simulink model "modl4"  (Simulink 4.00)
settings: Solver=ode45  StartTime=0.0  StopTime=2.0  RelTol=1e-4
libraries: simulink_extras x2
settings Model: BlockReductionOpt=off

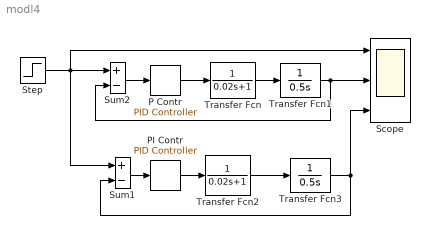
== system modl4 ==
  P Contr : simulink_extras/Additional Linear/PID Controller  P=12.5  I=0  D=0
  PI Contr : simulink_extras/Additional Linear/PID Controller  P=12.5  I=150  D=0.
  Scope : Scope  NumInputPorts=3
      settings: TimeRange=auto  YMin=-5~-5~-5  YMax=5~5~5  SaveToWorkspace=off  SaveName=ScopeData  MaxDataPoints=5000
  Step : Step  Time=0.1  Before=0  After=1  SampleTime=0
  Sum1 : Sum  Inputs=+-  SaturateOnIntegerOverflow=on
  Sum2 : Sum  Inputs=+-  SaturateOnIntegerOverflow=on
  Transfer Fcn : TransferFcn  Numerator=[1]  Denominator=[ 0.02 1]  Realization=auto  AbsoluteTolerance=auto
  Transfer Fcn1 : TransferFcn  Numerator=[1]  Denominator=[ 0.5 0]  Realization=auto  AbsoluteTolerance=auto
  Transfer Fcn2 : TransferFcn  Numerator=[1]  Denominator=[ 0.02 1]  Realization=auto  AbsoluteTolerance=auto
  Transfer Fcn3 : TransferFcn  Numerator=[1]  Denominator=[ 0.5 0]  Realization=auto  AbsoluteTolerance=auto
  wires:
  Step/1 -> Scope/1, Sum2/1, Sum1/1
  Sum1/1 -> PI Contr/1
  PI Contr/1 -> Transfer Fcn2/1
  Transfer Fcn/1 -> Transfer Fcn1/1
  Transfer Fcn1/1 -> Scope/2, Sum2/2
  P Contr/1 -> Transfer Fcn/1
  Sum2/1 -> P Contr/1
  Transfer Fcn2/1 -> Transfer Fcn3/1
  Transfer Fcn3/1 -> Sum1/2, Scope/3
